simulink model "gate_V25_2016a"  (R2016a)
settings: Solver=FixedStepAuto  StartTime=0.0  StopTime=100  FixedStep=0.001  RelTol=1e-3
values from neighbouring files (symbols this model uses):
  CLOSE_CHAR = CHAR_STAR    (= 42)    [GateParameter.m]
  CLOSE_SIDE_VALUE = 2.95*oneSec    (= 2950)    [GateParameter.m]
  CLOSED = 12    [GateParameter.m]
  CLOSING = 13    [GateParameter.m]
  NO_PASS_ASSIG = 6    [GateParameter.m]
  OPEN = 14    [GateParameter.m]
  OPEN_CHAR = CHAR_HASH    (= 35)    [GateParameter.m]
  OPEN_SIDE_VALUE = 3*oneSec    (= 3000)    [GateParameter.m]
  OPEN_TIMEOUT = 60*oneSec    (= 60000)    [GateParameter.m]
  OPENING = 11    [GateParameter.m]
  OPENING_ACTIVE = 1    [GateParameter.m]
  PASS_ASSIGNED = 7    [GateParameter.m]
  PASS_INCOMPLETE = 8    [GateParameter.m]
  PASS_TIMEOUT = 10*oneSec    (= 10000)    [GateParameter.m]
  PASSWORD_VERIFIED = 5    [GateParameter.m]
  TIMEOUT = 9    [GateParameter.m]
  WRONG_PASSWORD = 2    [GateParameter.m]
undefined symbols (not defined in the file or in its folder): sigbuilder_block
libraries: simulink x9, arduinolib x4
(part 1 of 3)
settings Model: ExtModeTrigDuration=2  Creator=omaro  LastModifiedBy=oelkawok
settings OptimizationCC: DefaultParameterBehavior=Inlined  InlineInvariantSignals=on  StateBitsets=on  DataBitsets=on  LifeSpan=1  MaxStackSize=64
settings DebuggingCC: UniqueDataStoreMsg=error  StrictBusMsg=ErrorOnBusTreatedAsVector
settings HardwareCC: ProdBitPerInt=16  ProdBitPerPointer=16  ProdLargestAtomicFloat=None  ProdWordSize=8  ProdHWDeviceType=Atmel->AVR
settings SFSimCC: SimCustomHeaderCode=|
  | //#include "C:\Users\omaro\Desktop\Gate_Model\Arduino\Arduino.h"
  | //#include "Keypad\Keypad.h"
settings RTWCC: SystemTargetFile=ert.tlc  HardwareBoard=Arduino Nano 3.0  TLCOptions=-aInlineSetEventsForThisBaseRateFcn=TLC_FALSE -aSuppressMultiTaskScheduler=TLC_FALSE -aRateBasedStepFcn=1  TemplateMakefile=ert_default_tmf  GenerateReport=on  RTWUseSimCustomCode=on  Toolchain=Arduino AVR v1.6.1  BuildConfiguration=Faster Runs  LaunchReport=on
settings RTWCC: CustomHeaderCode=|
  | //#include "C:\Users\omaro\Desktop\Gate_Model\Arduino\Arduino.h"
  | //#include "Keypad\Keypad.h"
settings CodeAppCC: ForceParamTrailComments=on  OperatorAnnotations=on  MATLABSourceComments=on
settings ERTTargetCC: ERTCustomFileBanners=off  SupportContinuousTime=on  SupportNonInlinedSFcns=on  SupportVariableSizeSignals=on  ModelStepFunctionPrototypeControlCompliant=off  RootIOFormat=Structure reference

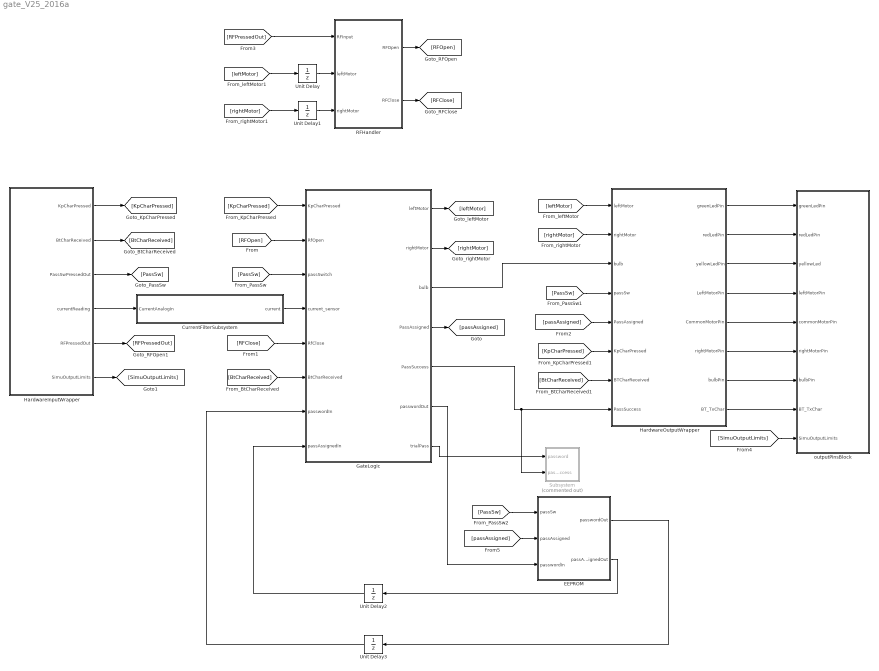
== system gate_V25_2016a ==
  CurrentFilterSubsystem : Subsystem
  EEPROM : Subsystem
  GateLogic : Subsystem  Variant=on  VariantControl=Variant1  OverrideUsingVariant=Variant2
  HardwareInputWrapper : Subsystem  Variant=on  VariantControl=Variant1  OverrideUsingVariant=Variant
  HardwareOutputWrapper : Subsystem  Variant=on  VariantControl=Variant1  OverrideUsingVariant=Variant2
  RFHandler : Subsystem
  Subsystem : Subsystem  Commented=on
  Unit Delay{,1..3} (4 alike) : UnitDelay  SampleTime=-1
  outputPinsBlock : Subsystem  Variant=on  VariantControl=Variant1  OverrideUsingVariant=Variant1
  wires:
  RFHandler/1(RFOpen) -> [RFOpen]
  RFHandler/2(RFClose) -> [RFClose]
  [RFPressedOut] -> RFHandler/1(RFInput)
  HardwareInputWrapper/5(RFPressedOut) -> [RFPressedOut]
  HardwareInputWrapper/3(PassSwPressedOut) -> [PassSw]
  [leftMotor] -> Unit Delay/1
  Unit Delay/1 -> RFHandler/2(leftMotor)
  [rightMotor] -> Unit Delay1/1
  Unit Delay1/1 -> RFHandler/3(rightMotor)
  HardwareInputWrapper/2(BtCharReceived) -> [BtCharReceived]
  HardwareInputWrapper/6(SimuOutputLimits) -> [SimuOutputLimits]
  [SimuOutputLimits] -> outputPinsBlock/9(SimuOutputLimits)
  HardwareInputWrapper/1(KpCharPressed) -> [KpCharPressed]
  [RFOpen] -> GateLogic/2(RfOpen)
  [PassSw] -> GateLogic/3(passSwitch)
  HardwareInputWrapper/4(currentReading) -> CurrentFilterSubsystem/1(CurrentAnalogIn)
  [RFClose] -> GateLogic/5(RfClose)
  [BtCharReceived] -> GateLogic/6(BtCharReceived)
  GateLogic/1(leftMotor) -> [leftMotor]
  GateLogic/2(rightMotor) -> [rightMotor]
  [KpCharPressed] -> GateLogic/1(KpCharPressed)
  [leftMotor] -> HardwareOutputWrapper/1("leftMotor ")
  [rightMotor] -> HardwareOutputWrapper/2("rightMotor ")
  GateLogic/3(bulb) -> HardwareOutputWrapper/3("bulb ")
  [PassSw] -> HardwareOutputWrapper/4("passSw ")
  [KpCharPressed] -> HardwareOutputWrapper/6("KpCharPressed ")
  [BtCharReceived] -> HardwareOutputWrapper/7("BTCharReceived ")
  HardwareOutputWrapper/1(" greenLedPin") -> outputPinsBlock/1(greenLedPin)
  HardwareOutputWrapper/2(" redLedPin") -> outputPinsBlock/2(redLedPin)
  HardwareOutputWrapper/3(" yellowLedPin") -> outputPinsBlock/3(yellowLed)
  HardwareOutputWrapper/4(" LeftMotorPin") -> outputPinsBlock/4(leftMotorPin)
  HardwareOutputWrapper/5(" CommonMotorPin") -> outputPinsBlock/5(commonMotorPin)
  HardwareOutputWrapper/6(" rightMotorPin") -> outputPinsBlock/6(rightMotorPin)
  HardwareOutputWrapper/7(" bulbPin") -> outputPinsBlock/7(bulbPin)
  HardwareOutputWrapper/8(" BT_TxChar") -> outputPinsBlock/8(BT_TxChar)
  GateLogic/4(PassAssigned) -> [passAssigned]
  [passAssigned] -> HardwareOutputWrapper/5("PassAssigned ")
  [passAssigned] -> EEPROM/2(passAssigned)
  [PassSw] -> EEPROM/1(passSw)
  GateLogic/6(passwordOut) -> EEPROM/3(passwordIn)
  EEPROM/1(passwordOut) -> Unit Delay3/1
  EEPROM/2(passAssignedOut) -> Unit Delay2/1
  Unit Delay2/1 -> GateLogic/8(passAssignedIn)
  Unit Delay3/1 -> GateLogic/7(passwordIn)
  GateLogic/5(PassSuccess) -> Subsystem/2(passSuccess), HardwareOutputWrapper/8("PassSuccess ")
  GateLogic/7(trialPass) -> Subsystem/1(password)
  CurrentFilterSubsystem/1(current) -> GateLogic/4(current_sensor)

== system gate_V25_2016a/CurrentFilterSubsystem ==
  CurrentAnalogIn : Inport
  10msSmapler : Stateflow chart  TreatAsAtomicUnit=on
      settings: PermitHierarchicalResolution=ParametersOnly
  Subsystem : Subsystem
  current : Outport
  wires:
  CurrentAnalogIn/1 -> Subsystem/1(CurrentAnalogIn)
  Subsystem/1(current) -> current/1
  10msSmapler/1(triggerOn()) -> Subsystem/Trigger

== system gate_V25_2016a/EEPROM ==
  passSw : Inport
  passAssigned : Inport  Port=2
  passwordIn : Inport  Port=3
  EEPROM_Control : Stateflow chart  TreatAsAtomicUnit=on
      settings: PermitHierarchicalResolution=ParametersOnly
  EEPROM_UPDATE : Subsystem  TreatAsAtomicUnit=on
  Subsystem2 : Subsystem  Commented=on
  Unit Delay : UnitDelay  SampleTime=-1
  Unit Delay1 : UnitDelay  SampleTime=-1
  passwordOut : Outport
  passAssignedOut : Outport  Port=2
  wires:
  passSw/1 -> EEPROM_Control/1(passSw)
  Unit Delay/1 -> EEPROM_Control/3(readComplete)
  Unit Delay1/1 -> EEPROM_Control/4(writeComplete)
  EEPROM_Control/1(clearReq) -> EEPROM_UPDATE/1(clearReq)
  EEPROM_Control/2(readReq) -> EEPROM_UPDATE/2(readReq)
  EEPROM_Control/3(writeReq) -> EEPROM_UPDATE/3(writeReq)
  passwordIn/1 -> EEPROM_UPDATE/4(passwordIn)
  [passAssigned] -> EEPROM_Control/2(passAssigned)
  [passAssigned] -> EEPROM_UPDATE/5(passAssignedIn)
  passAssigned/1 -> [passAssigned]
  EEPROM_UPDATE/1(readComplete) -> [readComplete]
  [readComplete] -> Unit Delay/1
  [writeComplete] -> Unit Delay1/1
  EEPROM_UPDATE/2(writeComplete) -> [writeComplete]
  EEPROM_UPDATE/4(passwordOut) -> passwordOut/1
  EEPROM_UPDATE/5(passAssignedOut) -> passAssignedOut/1

== system gate_V25_2016a/GateLogic ==
  KpCharPressed : Inport
  RfOpen : Inport  Port=2
  passSwitch : Inport  Port=3
  current_sensor : Inport  Port=4
  RfClose : Inport  Port=5
  BtCharReceived : Inport  Port=6
  passwordIn : Inport  Port=7
  passAssignedIn : Inport  Port=8
  A_Variant_BT_KP_RF : Subsystem  VariantControl=Variant
  B_Variant_KP_RF : Subsystem  VariantControl=Variant2
  C_Variant_RF : Subsystem  VariantControl=Variant3
  leftMotor : Outport
  rightMotor : Outport  Port=2
  bulb : Outport  Port=3
  PassAssigned : Outport  Port=4
  PassSuccess : Outport  Port=5
  passwordOut : Outport  Port=6
  trialPass : Outport  Port=7

== system gate_V25_2016a/HardwareInputWrapper ==
  HIL : Subsystem  VariantControl=Variant2
  MIL : Subsystem  VariantControl=Variant
  KpCharPressed : Outport
  BtCharReceived : Outport  Port=2
  PassSwPressedOut : Outport  Port=3
  currentReading : Outport  Port=4
  RFPressedOut : Outport  Port=5
  SimuOutputLimits : Outport  Port=6

== system gate_V25_2016a/HardwareOutputWrapper ==
  "leftMotor " : Inport
  "rightMotor " : Inport  Port=2
  "bulb " : Inport  Port=3
  "passSw " : Inport  Port=4
  "PassAssigned " : Inport  Port=5
  "KpCharPressed " : Inport  Port=6
  "BTCharReceived " : Inport  Port=7
  "PassSuccess " : Inport  Port=8
  A_HardwareOutputWrapper_BT_KP_RF : Subsystem  VariantControl=Variant1
  B_HardwareOutputWrapper_KP_RF : Subsystem  VariantControl=Variant2
  C_HardwareOutputWrapper_RF : Subsystem  VariantControl=Variant3
  " greenLedPin" : Outport
  " redLedPin" : Outport  Port=2
  " yellowLedPin" : Outport  Port=3
  " LeftMotorPin" : Outport  Port=4
  " CommonMotorPin" : Outport  Port=5
  " rightMotorPin" : Outport  Port=6
  " bulbPin" : Outport  Port=7
  " BT_TxChar" : Outport  Port=8

== system gate_V25_2016a/RFHandler ==
  RFInput : Inport
  leftMotor : Inport  Port=2
  rightMotor : Inport  Port=3
  CLOSED : Constant  Value=CLOSED  SampleTime=-1
  CLOSING : Constant  Value=CLOSING  SampleTime=-1
  OPEN : Constant  Value=OPEN  SampleTime=-1
  OPENING : Constant  Value=OPENING  SampleTime=-1
  RFHandlerL : Stateflow chart  TreatAsAtomicUnit=on
      settings: PermitHierarchicalResolution=ParametersOnly
  Scope : Scope
  RFOpen : Outport
  RFClose : Outport  Port=2
  wires:
  RFInput/1 -> RFHandlerL/1(btn)
  RFHandlerL/1(RFClose) -> RFClose/1
  RFHandlerL/2(RFOpen) -> Scope/1, RFOpen/1
  OPEN/1 -> RFHandlerL/6(OPEN)
  CLOSING/1 -> RFHandlerL/5(CLOSING)
  CLOSED/1 -> RFHandlerL/4(CLOSED)
  OPENING/1 -> RFHandlerL/7(OPENING)
  leftMotor/1 -> RFHandlerL/2(leftMotor)
  rightMotor/1 -> RFHandlerL/3(rightMotor)

== system gate_V25_2016a/Subsystem ==
  password : Inport
  passSuccess : Inport  Port=2
  S-Function Builder1 : S-Function  Commented=on  InitFcn=try, set_param(gcb,'FunctionName','printingBlock'), end  FunctionName=printingBlock  SFunctionModules=printingBlock_wrapper  SFunctionDeploymentMode=off  EnableBusSupport=off  mask(S-Function Builder){}
      mask help: Simulink:masks:SFunctionBuilder_MD
      mask init:
      | val = [[.9  0.75 0.75 1 1 .9 .9 1]',[1 1 0.75 0.75 .9 .9 1 .9]'];try , sys = get_param(gcb,'SfunBuilderFcnName');if isempty(sys), sys = get_param(gcb,'FunctionName'); end,catch, sys = get_param(gcb,'FunctionName'); end
      settings: CopyFcn=set_param(gcbh,'LinkStatus','none')  PreSaveFcn=try, set_param(gcb,'FunctionName','printingBlock'), end  OpenFcn=sfunctionwizard(gcbh)
      mask Display: plot(val(:,1),val(:,2)),disp(sys), port_label('input',1,'input'), port_label('input',2,'oldInput')
  S-Function Builder2 : S-Function  InitFcn=try, set_param(gcb,'FunctionName','printingPassBlock'), end  FunctionName=printingPassBlock  SFunctionModules=printingPassBlock_wrapper  SFunctionDeploymentMode=off  EnableBusSupport=off  mask(S-Function Builder){}
      mask help: Simulink:masks:SFunctionBuilder_MD
      mask init: same as gate_V25_2016a/Subsystem/S-Function Builder1
      settings: CopyFcn=set_param(gcbh,'LinkStatus','none')  PreSaveFcn=try, set_param(gcb,'FunctionName','printingPassBlock'), end  OpenFcn=sfunctionwizard(gcbh)
      mask Display: plot(val(:,1),val(:,2)),disp(sys), port_label('input',1,'password'), port_label('input',2,'passSuccess')
  wires:
  password/1 -> S-Function Builder2/1
  passSuccess/1 -> S-Function Builder2/2

== system gate_V25_2016a/outputPinsBlock ==
  greenLedPin : Inport
  redLedPin : Inport  Port=2
  yellowLed : Inport  Port=3
  leftMotorPin : Inport  Port=4
  commonMotorPin : Inport  Port=5
  rightMotorPin : Inport  Port=6
  bulbPin : Inport  Port=7
  BT_TxChar : Inport  Port=8
  SimuOutputLimits : Inport  Port=9
  HIL : Subsystem  VariantControl=Variant
  MIL : Subsystem  Variant=on  VariantControl=Variant1  OverrideUsingVariant=Variant1

== system gate_V25_2016a/CurrentFilterSubsystem/Subsystem ==
  CurrentAnalogIn : Inport
  Trigger : TriggerPort  TriggerType=function-call  VariantControl=Variant  PortDimensions=1
  Scope : Scope
  SquareWaveDetector : Stateflow chart  TreatAsAtomicUnit=on
      settings: PermitHierarchicalResolution=ParametersOnly
  Unit Delay : UnitDelay  SampleTime=-1
  current : Outport
  wires:
  Unit Delay/1 -> SquareWaveDetector/2(CurrentAnalogInOld)
  CurrentAnalogIn/1 -> Unit Delay/1, SquareWaveDetector/1(CurrentAnalogIn)
  SquareWaveDetector/1(currentValue) -> current/1, Scope/1

== system gate_V25_2016a/EEPROM/EEPROM_UPDATE ==
  clearReq : Inport
  readReq : Inport  Port=2
  writeReq : Inport  Port=3
  passwordIn : Inport  Port=4
  passAssignedIn : Inport  Port=5
  S-Function Builder : S-Function  InitFcn=try, set_param(gcb,'FunctionName','myEEPROM_Handler'), end  FunctionName=myEEPROM_Handler  SFunctionModules=myEEPROM_Handler_wrapper  SFunctionDeploymentMode=off  EnableBusSupport=off  mask(S-Function Builder){}
      mask help: Simulink:masks:SFunctionBuilder_MD
      mask init: same as gate_V25_2016a/Subsystem/S-Function Builder1
      settings: CopyFcn=set_param(gcbh,'LinkStatus','none')  PreSaveFcn=try, set_param(gcb,'FunctionName','myEEPROM_Handler'), end  OpenFcn=sfunctionwizard(gcbh)
      mask Display: plot(val(:,1),val(:,2)),disp(sys), port_label('input',1,'passwordIn'), port_label('input',2,'readReq'), port_label('input',3,'oldReadReq'), port_label('input',4,'clearReq'), port_label('input',5,'oldClearReq'), port_label('input',6,'writeReq'), port_label('input',7,'oldWriteReq'), port_label('input',8,'passAssignedIn'), port_label('output',1,'passwordOut'), port_label('output',2,'readComplete'), port_label('output',3,'writeComplete'), port_label('output',4,'clearComplete'), port_label('output',5,'passAssignedOut')
  Unit Delay : UnitDelay  SampleTime=-1
  Unit Delay1 : UnitDelay  SampleTime=-1
  Unit Delay2 : UnitDelay  SampleTime=-1
  readComplete : Outport
  writeComplete : Outport  Port=2
  clearComplete : Outport  Port=3
  passwordOut : Outport  Port=4
  passAssignedOut : Outport  Port=5
  wires:
  S-Function Builder/3 -> writeComplete/1
  S-Function Builder/2 -> readComplete/1
  S-Function Builder/4 -> clearComplete/1
  passwordIn/1 -> S-Function Builder/1
  readReq/1 -> Unit Delay/1, S-Function Builder/2
  Unit Delay/1 -> S-Function Builder/3
  clearReq/1 -> Unit Delay1/1, S-Function Builder/4
  passAssignedIn/1 -> S-Function Builder/8
  writeReq/1 -> Unit Delay2/1, S-Function Builder/6
  Unit Delay2/1 -> S-Function Builder/7
  Unit Delay1/1 -> S-Function Builder/5
  S-Function Builder/1 -> passwordOut/1
  S-Function Builder/5 -> passAssignedOut/1

== system gate_V25_2016a/EEPROM/Subsystem2 ==
  clearReq : Inport
  readReq : Inport  Port=2
  writeReq : Inport  Port=3
  passwordIn : Inport  Port=4
  passAssignedIn : Inport  Port=5
  S-Function Builder : S-Function  InitFcn=try, set_param(gcb,'FunctionName','EEPROM_Handler'), end  FunctionName=EEPROM_Handler  SFunctionModules=EEPROM_Handler_wrapper  SFunctionDeploymentMode=off  EnableBusSupport=off  mask(S-Function Builder){}
      mask help: Simulink:masks:SFunctionBuilder_MD
      mask init: same as gate_V25_2016a/Subsystem/S-Function Builder1
      settings: CopyFcn=set_param(gcbh,'LinkStatus','none')  PreSaveFcn=try, set_param(gcb,'FunctionName','EEPROM_Handler'), end  OpenFcn=sfunctionwizard(gcbh)
      mask Display:
      | plot(val(:,1),val(:,2))
      | disp(sys)
      | port_label('input',1,'passwordIn')
      | port_label('input',2,'readReq')
      | port_label('input',3,'clearReq')
      | port_label('input',4,'writeReq')
      | port_label('input',5,'passAssignedIn')
      | port_label('output',1,'passwordOut')
      | port_label('output',2,'readComplete')
      | port_label('output',3,'writeComplete')
      | port_label('output',4,'clearComplete')
      | port_label('output',5,'passAssignedOut')
  Scope3 : Scope  NumInputPorts=5
  readComplete : Outport
  writeComplete : Outport  Port=2
  clearComplete : Outport  Port=3
  passwordOut : Outport  Port=4
  passAssignedOut : Outport  Port=5
  wires:
  S-Function Builder/5 -> passAssignedOut/1, Scope3/5
  S-Function Builder/3 -> writeComplete/1, Scope3/3
  S-Function Builder/2 -> readComplete/1, Scope3/2
  S-Function Builder/1 -> passwordOut/1, Scope3/1
  S-Function Builder/4 -> clearComplete/1, Scope3/4
  passAssignedIn/1 -> S-Function Builder/5
  clearReq/1 -> S-Function Builder/3
  passwordIn/1 -> S-Function Builder/1
  readReq/1 -> S-Function Builder/2
  writeReq/1 -> S-Function Builder/4

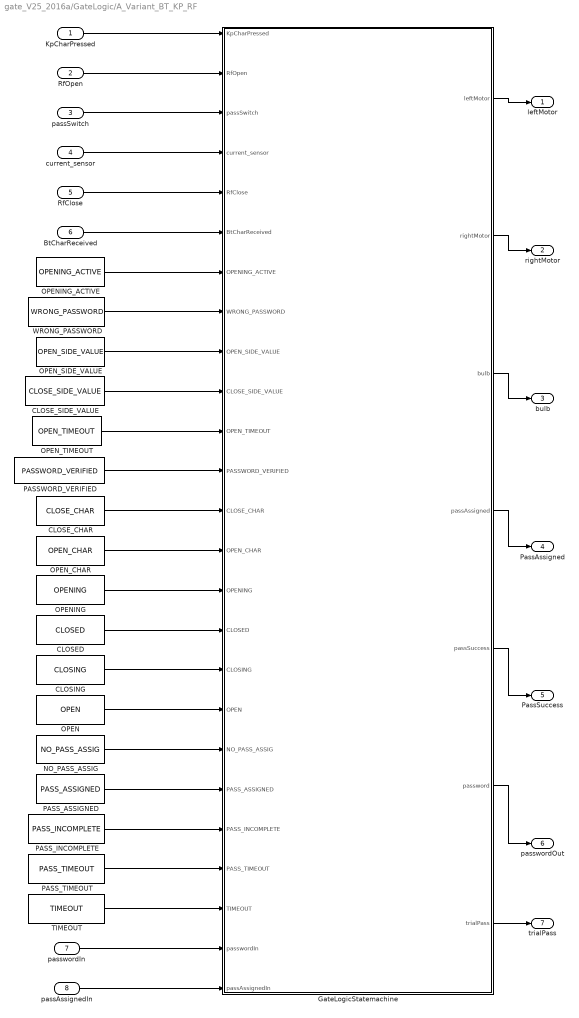
== system gate_V25_2016a/GateLogic/A_Variant_BT_KP_RF ==
  KpCharPressed : Inport
  RfOpen : Inport  Port=2
  passSwitch : Inport  Port=3
  current_sensor : Inport  Port=4
  RfClose : Inport  Port=5
  BtCharReceived : Inport  Port=6
  passwordIn : Inport  Port=7
  passAssignedIn : Inport  Port=8
  CLOSED : Constant  Value=CLOSED  SampleTime=-1
  CLOSE_CHAR : Constant  Value=CLOSE_CHAR  SampleTime=-1
  CLOSE_SIDE_VALUE : Constant  Value=CLOSE_SIDE_VALUE  SampleTime=-1
  CLOSING : Constant  Value=CLOSING  SampleTime=-1
  GateLogicStatemachine : Stateflow chart  TreatAsAtomicUnit=on
      settings: PermitHierarchicalResolution=ParametersOnly
  NO_PASS_ASSIG : Constant  Value=NO_PASS_ASSIG  SampleTime=-1
  OPEN : Constant  Value=OPEN  SampleTime=-1
  OPENING : Constant  Value=OPENING  SampleTime=-1
  OPENING_ACTIVE : Constant  Value=OPENING_ACTIVE  SampleTime=-1
  OPEN_CHAR : Constant  Value=OPEN_CHAR  SampleTime=-1
  OPEN_SIDE_VALUE : Constant  Value=OPEN_SIDE_VALUE  SampleTime=-1
  OPEN_TIMEOUT : Constant  Value=OPEN_TIMEOUT  SampleTime=-1
  PASSWORD_VERIFIED : Constant  Value=PASSWORD_VERIFIED  SampleTime=-1
  PASS_ASSIGNED : Constant  Value=PASS_ASSIGNED  SampleTime=-1
  PASS_INCOMPLETE : Constant  Value=PASS_INCOMPLETE  SampleTime=-1
  PASS_TIMEOUT : Constant  Value=PASS_TIMEOUT  SampleTime=-1
  TIMEOUT : Constant  Value=TIMEOUT  SampleTime=-1
  WRONG_PASSWORD : Constant  Value=WRONG_PASSWORD  SampleTime=-1
  leftMotor : Outport
  rightMotor : Outport  Port=2
  bulb : Outport  Port=3
  PassAssigned : Outport  Port=4
  PassSuccess : Outport  Port=5
  passwordOut : Outport  Port=6
  trialPass : Outport  Port=7
  wires:
  RfClose/1 -> GateLogicStatemachine/5(RfClose)
  TIMEOUT/1 -> GateLogicStatemachine/23(TIMEOUT)
  PASS_INCOMPLETE/1 -> GateLogicStatemachine/21(PASS_INCOMPLETE)
  PASS_ASSIGNED/1 -> GateLogicStatemachine/20(PASS_ASSIGNED)
  GateLogicStatemachine/4(passAssigned) -> PassAssigned/1
  passSwitch/1 -> GateLogicStatemachine/3(passSwitch)
  GateLogicStatemachine/5(passSuccess) -> PassSuccess/1
  PASS_TIMEOUT/1 -> GateLogicStatemachine/22(PASS_TIMEOUT)
  KpCharPressed/1 -> GateLogicStatemachine/1(KpCharPressed)
  BtCharReceived/1 -> GateLogicStatemachine/6(BtCharReceived)
  NO_PASS_ASSIG/1 -> GateLogicStatemachine/19(NO_PASS_ASSIG)
  CLOSE_SIDE_VALUE/1 -> GateLogicStatemachine/10(CLOSE_SIDE_VALUE)
  OPEN_TIMEOUT/1 -> GateLogicStatemachine/11(OPEN_TIMEOUT)
  OPEN_SIDE_VALUE/1 -> GateLogicStatemachine/9(OPEN_SIDE_VALUE)
  OPENING_ACTIVE/1 -> GateLogicStatemachine/7(OPENING_ACTIVE)
  GateLogicStatemachine/2(rightMotor) -> rightMotor/1
  GateLogicStatemachine/1(leftMotor) -> leftMotor/1
  WRONG_PASSWORD/1 -> GateLogicStatemachine/8(WRONG_PASSWORD)
  current_sensor/1 -> GateLogicStatemachine/4(current_sensor)
  GateLogicStatemachine/3(bulb) -> bulb/1
  RfOpen/1 -> GateLogicStatemachine/2(RfOpen)
  PASSWORD_VERIFIED/1 -> GateLogicStatemachine/12(PASSWORD_VERIFIED)
  OPEN/1 -> GateLogicStatemachine/18(OPEN)
  CLOSE_CHAR/1 -> GateLogicStatemachine/13(CLOSE_CHAR)
  OPEN_CHAR/1 -> GateLogicStatemachine/14(OPEN_CHAR)
  CLOSED/1 -> GateLogicStatemachine/16(CLOSED)
  OPENING/1 -> GateLogicStatemachine/15(OPENING)
  CLOSING/1 -> GateLogicStatemachine/17(CLOSING)
  GateLogicStatemachine/6(password) -> passwordOut/1
  passwordIn/1 -> GateLogicStatemachine/24(passwordIn)
  passAssignedIn/1 -> GateLogicStatemachine/25(passAssignedIn)
  GateLogicStatemachine/7(trialPass) -> trialPass/1

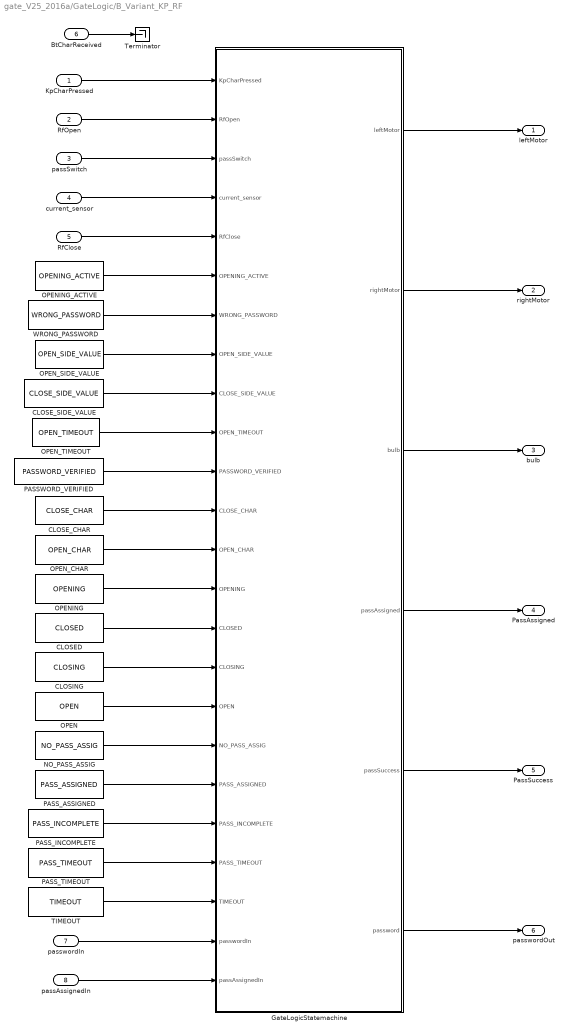
== system gate_V25_2016a/GateLogic/B_Variant_KP_RF ==
  KpCharPressed : Inport
  RfOpen : Inport  Port=2
  passSwitch : Inport  Port=3
  current_sensor : Inport  Port=4
  RfClose : Inport  Port=5
  BtCharReceived : Inport  Port=6
  passwordIn : Inport  Port=7
  passAssignedIn : Inport  Port=8
  CLOSED : Constant  Value=CLOSED  SampleTime=-1
  CLOSE_CHAR : Constant  Value=CLOSE_CHAR  SampleTime=-1
  CLOSE_SIDE_VALUE : Constant  Value=CLOSE_SIDE_VALUE  SampleTime=-1
  CLOSING : Constant  Value=CLOSING  SampleTime=-1
  GateLogicStatemachine : Stateflow chart  TreatAsAtomicUnit=on
      settings: PermitHierarchicalResolution=ParametersOnly
  NO_PASS_ASSIG : Constant  Value=NO_PASS_ASSIG  SampleTime=-1
  OPEN : Constant  Value=OPEN  SampleTime=-1
  OPENING : Constant  Value=OPENING  SampleTime=-1
  OPENING_ACTIVE : Constant  Value=OPENING_ACTIVE  SampleTime=-1
  OPEN_CHAR : Constant  Value=OPEN_CHAR  SampleTime=-1
  OPEN_SIDE_VALUE : Constant  Value=OPEN_SIDE_VALUE  SampleTime=-1
  OPEN_TIMEOUT : Constant  Value=OPEN_TIMEOUT  SampleTime=-1
  PASSWORD_VERIFIED : Constant  Value=PASSWORD_VERIFIED  SampleTime=-1
  PASS_ASSIGNED : Constant  Value=PASS_ASSIGNED  SampleTime=-1
  PASS_INCOMPLETE : Constant  Value=PASS_INCOMPLETE  SampleTime=-1
  PASS_TIMEOUT : Constant  Value=PASS_TIMEOUT  SampleTime=-1
  TIMEOUT : Constant  Value=TIMEOUT  SampleTime=-1
  Terminator : Terminator
  WRONG_PASSWORD : Constant  Value=WRONG_PASSWORD  SampleTime=-1
  leftMotor : Outport
  rightMotor : Outport  Port=2
  bulb : Outport  Port=3
  PassAssigned : Outport  Port=4
  PassSuccess : Outport  Port=5
  passwordOut : Outport  Port=6
  wires:
  CLOSING/1 -> GateLogicStatemachine/16(CLOSING)
  OPENING/1 -> GateLogicStatemachine/14(OPENING)
  CLOSED/1 -> GateLogicStatemachine/15(CLOSED)
  OPEN_CHAR/1 -> GateLogicStatemachine/13(OPEN_CHAR)
  CLOSE_CHAR/1 -> GateLogicStatemachine/12(CLOSE_CHAR)
  OPEN/1 -> GateLogicStatemachine/17(OPEN)
  PASSWORD_VERIFIED/1 -> GateLogicStatemachine/11(PASSWORD_VERIFIED)
  RfOpen/1 -> GateLogicStatemachine/2(RfOpen)
  GateLogicStatemachine/3(bulb) -> bulb/1
  current_sensor/1 -> GateLogicStatemachine/4(current_sensor)
  WRONG_PASSWORD/1 -> GateLogicStatemachine/7(WRONG_PASSWORD)
  GateLogicStatemachine/1(leftMotor) -> leftMotor/1
  GateLogicStatemachine/2(rightMotor) -> rightMotor/1
  OPENING_ACTIVE/1 -> GateLogicStatemachine/6(OPENING_ACTIVE)
  OPEN_SIDE_VALUE/1 -> GateLogicStatemachine/8(OPEN_SIDE_VALUE)
  OPEN_TIMEOUT/1 -> GateLogicStatemachine/10(OPEN_TIMEOUT)
  CLOSE_SIDE_VALUE/1 -> GateLogicStatemachine/9(CLOSE_SIDE_VALUE)
  NO_PASS_ASSIG/1 -> GateLogicStatemachine/18(NO_PASS_ASSIG)
  KpCharPressed/1 -> GateLogicStatemachine/1(KpCharPressed)
  PASS_TIMEOUT/1 -> GateLogicStatemachine/21(PASS_TIMEOUT)
  GateLogicStatemachine/5(passSuccess) -> PassSuccess/1
  passSwitch/1 -> GateLogicStatemachine/3(passSwitch)
  GateLogicStatemachine/4(passAssigned) -> PassAssigned/1
  PASS_ASSIGNED/1 -> GateLogicStatemachine/19(PASS_ASSIGNED)
  PASS_INCOMPLETE/1 -> GateLogicStatemachine/20(PASS_INCOMPLETE)
  TIMEOUT/1 -> GateLogicStatemachine/22(TIMEOUT)
  RfClose/1 -> GateLogicStatemachine/5(RfClose)
  BtCharReceived/1 -> Terminator/1
  passwordIn/1 -> GateLogicStatemachine/23(passwordIn)
  passAssignedIn/1 -> GateLogicStatemachine/24(passAssignedIn)
  GateLogicStatemachine/6(password) -> passwordOut/1

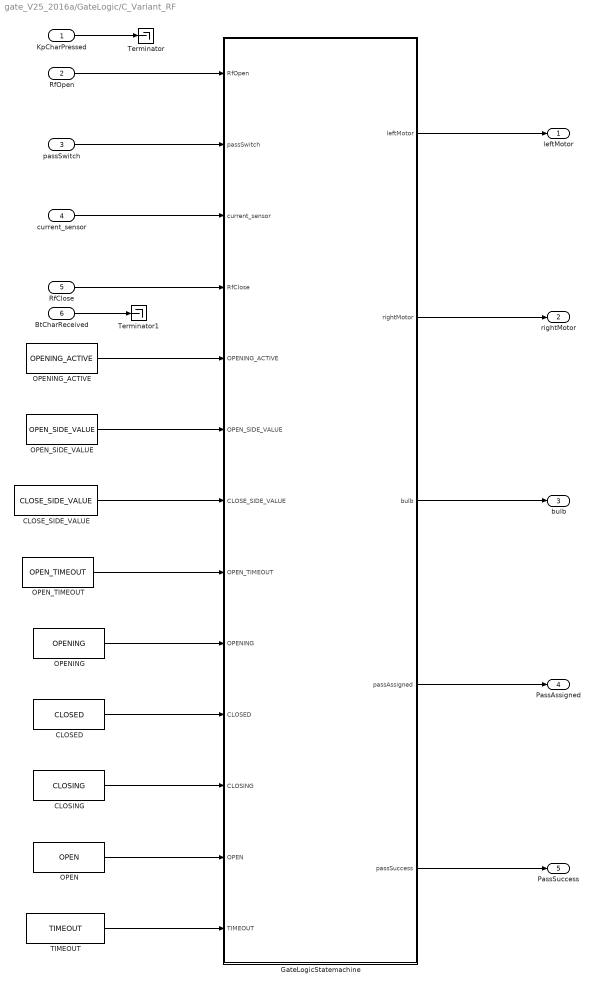
== system gate_V25_2016a/GateLogic/C_Variant_RF ==
  KpCharPressed : Inport
  RfOpen : Inport  Port=2
  passSwitch : Inport  Port=3
  current_sensor : Inport  Port=4
  RfClose : Inport  Port=5
  BtCharReceived : Inport  Port=6
  CLOSED : Constant  Value=CLOSED  SampleTime=-1
  CLOSE_SIDE_VALUE : Constant  Value=CLOSE_SIDE_VALUE  SampleTime=-1
  CLOSING : Constant  Value=CLOSING  SampleTime=-1
  GateLogicStatemachine : Stateflow chart  TreatAsAtomicUnit=on
      settings: PermitHierarchicalResolution=ParametersOnly
  OPEN : Constant  Value=OPEN  SampleTime=-1
  OPENING : Constant  Value=OPENING  SampleTime=-1
  OPENING_ACTIVE : Constant  Value=OPENING_ACTIVE  SampleTime=-1
  OPEN_SIDE_VALUE : Constant  Value=OPEN_SIDE_VALUE  SampleTime=-1
  OPEN_TIMEOUT : Constant  Value=OPEN_TIMEOUT  SampleTime=-1
  TIMEOUT : Constant  Value=TIMEOUT  SampleTime=-1
  Terminator : Terminator
  Terminator1 : Terminator
  leftMotor : Outport
  rightMotor : Outport  Port=2
  bulb : Outport  Port=3
  PassAssigned : Outport  Port=4
  PassSuccess : Outport  Port=5
  wires:
  RfClose/1 -> GateLogicStatemachine/4(RfClose)
  TIMEOUT/1 -> GateLogicStatemachine/13(TIMEOUT)
  GateLogicStatemachine/4(passAssigned) -> PassAssigned/1
  passSwitch/1 -> GateLogicStatemachine/2(passSwitch)
  GateLogicStatemachine/5(passSuccess) -> PassSuccess/1
  CLOSE_SIDE_VALUE/1 -> GateLogicStatemachine/7(CLOSE_SIDE_VALUE)
  OPEN_TIMEOUT/1 -> GateLogicStatemachine/8(OPEN_TIMEOUT)
  OPEN_SIDE_VALUE/1 -> GateLogicStatemachine/6(OPEN_SIDE_VALUE)
  OPENING_ACTIVE/1 -> GateLogicStatemachine/5(OPENING_ACTIVE)
  GateLogicStatemachine/2(rightMotor) -> rightMotor/1
  GateLogicStatemachine/1(leftMotor) -> leftMotor/1
  current_sensor/1 -> GateLogicStatemachine/3(current_sensor)
  GateLogicStatemachine/3(bulb) -> bulb/1
  RfOpen/1 -> GateLogicStatemachine/1(RfOpen)
  OPEN/1 -> GateLogicStatemachine/12(OPEN)
  CLOSED/1 -> GateLogicStatemachine/10(CLOSED)
  OPENING/1 -> GateLogicStatemachine/9(OPENING)
  CLOSING/1 -> GateLogicStatemachine/11(CLOSING)
  KpCharPressed/1 -> Terminator/1
  BtCharReceived/1 -> Terminator1/1

== system gate_V25_2016a/HardwareInputWrapper/HIL ==
  Analog Input : arduinolib/Analog Input  pinNumber=6  sampleTime=-1  blockPlatform=arduino
  BluetoothWrapper : Subsystem
  ButtonsPressed : Subsystem
  KeypadWrapper : Subsystem
  S-Function Builder1 : S-Function  Commented=on  InitFcn=try, set_param(gcb,'FunctionName','CurrentA_Lib'), end  FunctionName=CurrentA_Lib  SFunctionModules=CurrentA_Lib_wrapper  SFunctionDeploymentMode=off  EnableBusSupport=off  mask(S-Function Builder){}
      mask help: Simulink:masks:SFunctionBuilder_MD
      mask init: same as gate_V25_2016a/Subsystem/S-Function Builder1
      settings: CopyFcn=set_param(gcbh,'LinkStatus','none')  PreSaveFcn=try, set_param(gcb,'FunctionName','CurrentA_Lib'), end  OpenFcn=sfunctionwizard(gcbh)
      mask Display: plot(val(:,1),val(:,2)),disp(sys), port_label('output',1,'currentValue')
  S-Function Builder2 : S-Function  Commented=on  InitFcn=try, set_param(gcb,'FunctionName','printingBlock'), end  FunctionName=printingBlock  SFunctionModules=printingBlock_wrapper  SFunctionDeploymentMode=off  EnableBusSupport=off  mask(S-Function Builder){}
      mask help: Simulink:masks:SFunctionBuilder_MD
      mask init: same as gate_V25_2016a/Subsystem/S-Function Builder1
      settings: CopyFcn=set_param(gcbh,'LinkStatus','none')  PreSaveFcn=try, set_param(gcb,'FunctionName','printingBlock'), end  OpenFcn=sfunctionwizard(gcbh)
      mask Display: plot(val(:,1),val(:,2)),disp(sys), port_label('input',1,'uint8ToPrint')
  currentSensorWrapperOld : Subsystem  Commented=on
  KpCharPressed : Outport
  BtCharReceived : Outport  Port=2
  PassSwPressedOut : Outport  Port=3
  currentReading : Outport  Port=4
  RFPressedOut : Outport  Port=5
  wires:
  BluetoothWrapper/1(bluetoothCharPressed) -> BtCharReceived/1
  Analog Input/1 -> currentReading/1  "motorCrrent"
  KeypadWrapper/1(charPressed) -> S-Function Builder2/1, KpCharPressed/1
  ButtonsPressed/2(SWPressed) -> PassSwPressedOut/1
  ButtonsPressed/1(RFPressed) -> RFPressedOut/1

== system gate_V25_2016a/HardwareInputWrapper/MIL ==
  Bus Creator : BusCreator  Inputs=16
  Quantizer{,1..3} (4 alike) : Quantizer  QuantizationInterval=-1
  Signal Builder : Subsystem  Tag=STV Subsys  LoadFcn=sigbuilder_block('load');  StartFcn=sigbuilder_block('start');  StopFcn=sigbuilder_block('stop');  ClipboardFcn=sigbuilder_block('clipboard');  mask(Sigbuilder block){}
      mask help: Simulink:masks:SigbuilderBlock_MD
      mask init:
      | if ~strcmp(get_param(bdroot(gcbh),'SimulationStatus'),'stopped') tuvar = sigbuilder_block('maskInit'); end
      settings: CopyFcn=sigbuilder_block('copy');  DeleteFcn=sigbuilder_block('delete');  ModelCloseFcn=sigbuilder_block('modelClose');  PreSaveFcn=sigbuilder_block('preSave');  PauseFcn=sigbuilder_block('pause');  ContinueFcn=sigbuilder_block('continue');  NameChangeFcn=sigbuilder_block('namechange');  OpenFcn=sigbuilder_block('open',[6 28.2 1012.8 484.8 ]);  CloseFcn=sigbuilder_block('close');
      mask Display: plot(0, 0, 100, 100,[2, 2, 32, 32, 2], [68, 8, 8, 68, 68],[32, 2], [38, 38], [32, 19, 2],[53, 60, 44], [32, 17, 17, 2],[16, 16, 31, 31]);txt = getActiveGroup(gcbh);text(2, 100, txt,'verticalAlignment', 'top');
  KpCharPressed : Outport
  BtCharReceived : Outport  Port=2
  PassSwPressedOut : Outport  Port=3
  RFPressedOut : Outport  Port=4
  currentReading : Outport  Port=5
  SimuOutputLimits : Outport  Port=6
  wires:
  Signal Builder/2(BT_input) -> Quantizer1/1
  Signal Builder/4(SW_input) -> Quantizer3/1
  Signal Builder/1(Kp_input) -> Quantizer/1
  Signal Builder/3(RF_input) -> Quantizer2/1
  Quantizer/1 -> KpCharPressed/1
  Quantizer1/1 -> BtCharReceived/1
  Quantizer2/1 -> RFPressedOut/1
  Quantizer3/1 -> PassSwPressedOut/1
  Bus Creator/1 -> SimuOutputLimits/1
  Signal Builder/16(GreenLedMax) -> Bus Creator/11  "GreenLedMax"
  Signal Builder/15(YellowLedMin) -> Bus Creator/10  "YellowLedMin"
  Signal Builder/17(GreenLedMin) -> Bus Creator/12  "GreenLedMin"
  Signal Builder/14(YellowLedMax) -> Bus Creator/9  "YellowLedMax"
  Signal Builder/18(BulbMax) -> Bus Creator/13  "BulbMax"
  Signal Builder/13(RedLedMin) -> Bus Creator/8  "RedLedMin"
  Signal Builder/19(BulbMin) -> Bus Creator/14  "BulbMin"
  Signal Builder/20(BT_outputMax) -> Bus Creator/15  "BT_outputMax"
  Signal Builder/12(RedLedMax) -> Bus Creator/7  "RedLedMax"
  Signal Builder/11(MCMin) -> Bus Creator/6  "MCMin"
  Signal Builder/10(MCMax) -> Bus Creator/5  "MCMax"
  Signal Builder/9(MRMin) -> Bus Creator/4  "MRMin"
  Signal Builder/8(MRMax) -> Bus Creator/3  "MRMax"
  Signal Builder/7(MLMin) -> Bus Creator/2  "MLMin"
  Signal Builder/6(MLMax) -> Bus Creator/1  "MLMax"
  Signal Builder/21(BT_outputMin) -> Bus Creator/16  "BT_outputMin"
  Signal Builder/5(currentReading_input) -> currentReading/1

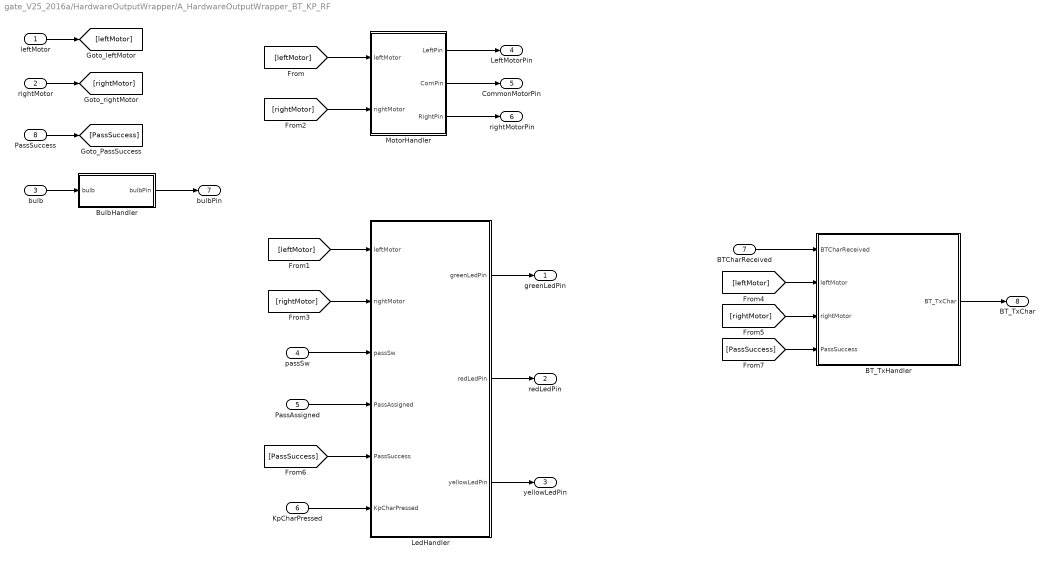
== system gate_V25_2016a/HardwareOutputWrapper/A_HardwareOutputWrapper_BT_KP_RF ==
  leftMotor : Inport
  rightMotor : Inport  Port=2
  bulb : Inport  Port=3
  passSw : Inport  Port=4
  PassAssigned : Inport  Port=5
  KpCharPressed : Inport  Port=6
  BTCharReceived : Inport  Port=7
  PassSuccess : Inport  Port=8
  BT_TxHandler : Subsystem
  BulbHandler : Subsystem
  LedHandler : Subsystem
  MotorHandler : Subsystem
  greenLedPin : Outport
  redLedPin : Outport  Port=2
  yellowLedPin : Outport  Port=3
  LeftMotorPin : Outport  Port=4
  CommonMotorPin : Outport  Port=5
  rightMotorPin : Outport  Port=6
  bulbPin : Outport  Port=7
  BT_TxChar : Outport  Port=8
  wires:
  [leftMotor] -> MotorHandler/1(leftMotor)
  [rightMotor] -> MotorHandler/2(rightMotor)
  bulb/1 -> BulbHandler/1(bulb)
  LedHandler/1(greenLedPin) -> greenLedPin/1
  LedHandler/2(redLedPin) -> redLedPin/1
  LedHandler/3(yellowLedPin) -> yellowLedPin/1
  MotorHandler/1(LeftPin) -> LeftMotorPin/1
  MotorHandler/2(ComPin) -> CommonMotorPin/1
  MotorHandler/3(RightPin) -> rightMotorPin/1
  BulbHandler/1(bulbPin) -> bulbPin/1
  leftMotor/1 -> [leftMotor]
  [leftMotor] -> LedHandler/1(leftMotor)
  rightMotor/1 -> [rightMotor]
  [rightMotor] -> LedHandler/2(rightMotor)
  passSw/1 -> LedHandler/3(passSw)
  PassAssigned/1 -> LedHandler/4(PassAssigned)
  [PassSuccess] -> LedHandler/5(PassSuccess)
  KpCharPressed/1 -> LedHandler/6(KpCharPressed)
  [leftMotor] -> BT_TxHandler/2(leftMotor)
  BTCharReceived/1 -> BT_TxHandler/1(BTCharReceived)
  [rightMotor] -> BT_TxHandler/3(rightMotor)
  PassSuccess/1 -> [PassSuccess]
  [PassSuccess] -> BT_TxHandler/4(PassSuccess)
  BT_TxHandler/1(BT_TxChar) -> BT_TxChar/1

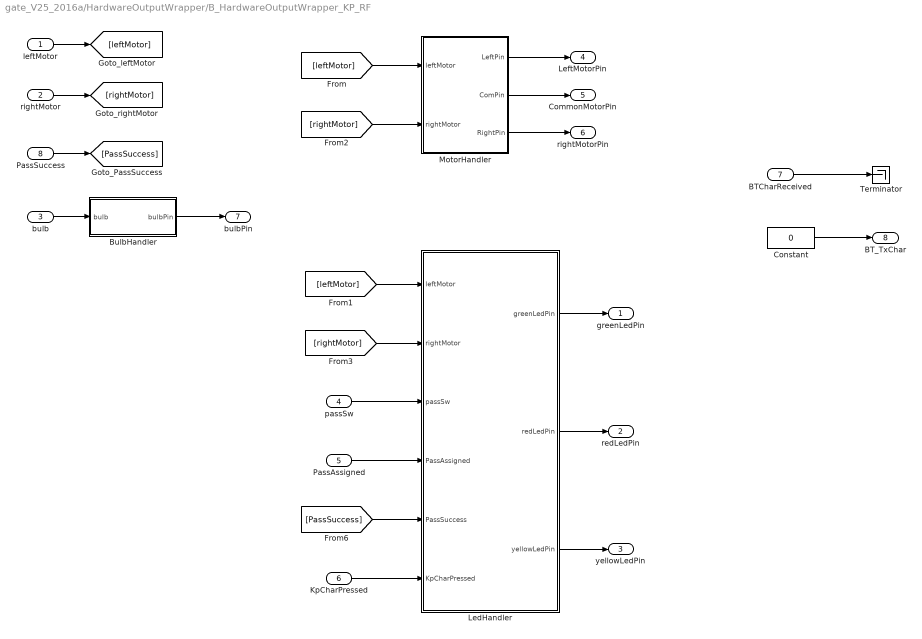
== system gate_V25_2016a/HardwareOutputWrapper/B_HardwareOutputWrapper_KP_RF ==
  leftMotor : Inport
  rightMotor : Inport  Port=2
  bulb : Inport  Port=3
  passSw : Inport  Port=4
  PassAssigned : Inport  Port=5
  KpCharPressed : Inport  Port=6
  BTCharReceived : Inport  Port=7
  PassSuccess : Inport  Port=8
  BulbHandler : Subsystem
  Constant : Constant  Value=0  SampleTime=-1
  LedHandler : Subsystem
  MotorHandler : Subsystem
  Terminator : Terminator
  greenLedPin : Outport
  redLedPin : Outport  Port=2
  yellowLedPin : Outport  Port=3
  LeftMotorPin : Outport  Port=4
  CommonMotorPin : Outport  Port=5
  rightMotorPin : Outport  Port=6
  bulbPin : Outport  Port=7
  BT_TxChar : Outport  Port=8
  wires:
  Constant/1 -> BT_TxChar/1
  PassSuccess/1 -> [PassSuccess]
  KpCharPressed/1 -> LedHandler/6(KpCharPressed)
  [PassSuccess] -> LedHandler/5(PassSuccess)
  PassAssigned/1 -> LedHandler/4(PassAssigned)
  passSw/1 -> LedHandler/3(passSw)
  [rightMotor] -> LedHandler/2(rightMotor)
  rightMotor/1 -> [rightMotor]
  [leftMotor] -> LedHandler/1(leftMotor)
  leftMotor/1 -> [leftMotor]
  BulbHandler/1(bulbPin) -> bulbPin/1
  MotorHandler/3(RightPin) -> rightMotorPin/1
  MotorHandler/2(ComPin) -> CommonMotorPin/1
  MotorHandler/1(LeftPin) -> LeftMotorPin/1
  LedHandler/3(yellowLedPin) -> yellowLedPin/1
  LedHandler/2(redLedPin) -> redLedPin/1
  LedHandler/1(greenLedPin) -> greenLedPin/1
  bulb/1 -> BulbHandler/1(bulb)
  [rightMotor] -> MotorHandler/2(rightMotor)
  [leftMotor] -> MotorHandler/1(leftMotor)
  BTCharReceived/1 -> Terminator/1

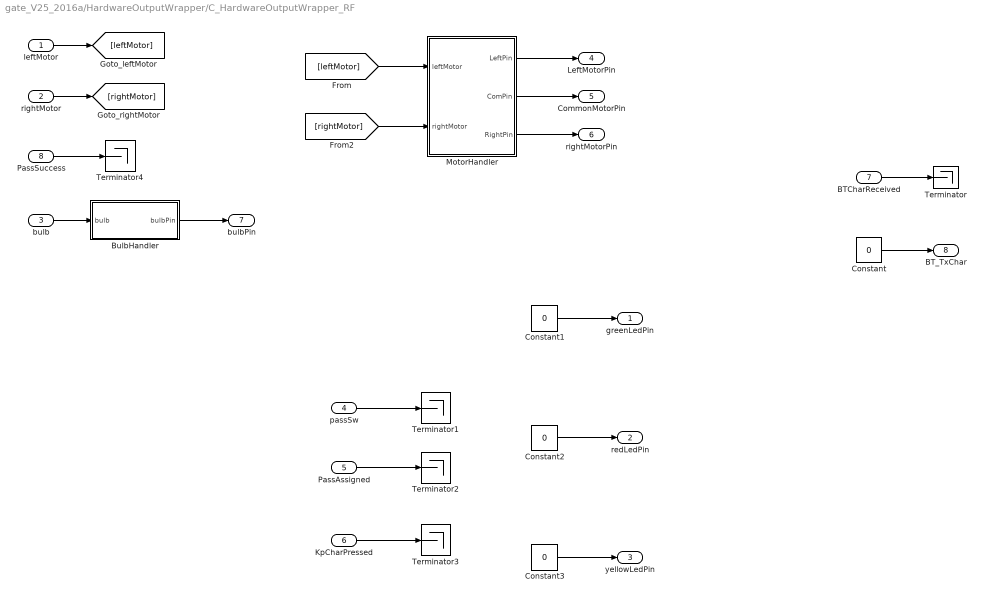
== system gate_V25_2016a/HardwareOutputWrapper/C_HardwareOutputWrapper_RF ==
  leftMotor : Inport
  rightMotor : Inport  Port=2
  bulb : Inport  Port=3
  passSw : Inport  Port=4
  PassAssigned : Inport  Port=5
  KpCharPressed : Inport  Port=6
  BTCharReceived : Inport  Port=7
  PassSuccess : Inport  Port=8
  BulbHandler : Subsystem
  Constant{,1..3} (4 alike) : Constant  Value=0  SampleTime=-1
  MotorHandler : Subsystem
  Terminator{,1..4} (5 alike) : Terminator
  greenLedPin : Outport
  redLedPin : Outport  Port=2
  yellowLedPin : Outport  Port=3
  LeftMotorPin : Outport  Port=4
  CommonMotorPin : Outport  Port=5
  rightMotorPin : Outport  Port=6
  bulbPin : Outport  Port=7
  BT_TxChar : Outport  Port=8
  wires:
  [leftMotor] -> MotorHandler/1(leftMotor)
  [rightMotor] -> MotorHandler/2(rightMotor)
  bulb/1 -> BulbHandler/1(bulb)
  MotorHandler/1(LeftPin) -> LeftMotorPin/1
  MotorHandler/2(ComPin) -> CommonMotorPin/1
  MotorHandler/3(RightPin) -> rightMotorPin/1
  BulbHandler/1(bulbPin) -> bulbPin/1
  leftMotor/1 -> [leftMotor]
  rightMotor/1 -> [rightMotor]
  PassSuccess/1 -> Terminator4/1
  BTCharReceived/1 -> Terminator/1
  Constant/1 -> BT_TxChar/1
  Constant3/1 -> yellowLedPin/1
  Constant2/1 -> redLedPin/1
  Constant1/1 -> greenLedPin/1
  passSw/1 -> Terminator1/1
  PassAssigned/1 -> Terminator2/1
  KpCharPressed/1 -> Terminator3/1

== system gate_V25_2016a/outputPinsBlock/HIL ==
  greenLedPin : Inport
  redLedPin : Inport  Port=2
  yellowLed : Inport  Port=3
  leftMotorPin : Inport  Port=4
  commonMotorPin : Inport  Port=5
  rightMotorPin : Inport  Port=6
  bulbPin : Inport  Port=7
  Digital Output : arduinolib/Digital Output  pinNumber=11  blockPlatform=arduino
  Digital Output1 : arduinolib/Digital Output  pinNumber=12  blockPlatform=arduino
  Digital Output2 : arduinolib/Digital Output  pinNumber=13  blockPlatform=arduino
  S-Function Builder1 : S-Function  InitFcn=try, set_param(gcb,'FunctionName','A2PIN_Lib'), end  FunctionName=A2PIN_Lib  SFunctionModules=A2PIN_Lib_wrapper  SFunctionDeploymentMode=off  EnableBusSupport=off  mask(S-Function Builder){}
      mask help: Simulink:masks:SFunctionBuilder_MD
      mask init: same as gate_V25_2016a/Subsystem/S-Function Builder1
      settings: CopyFcn=set_param(gcbh,'LinkStatus','none')  PreSaveFcn=try, set_param(gcb,'FunctionName','A2PIN_Lib'), end  OpenFcn=sfunctionwizard(gcbh)
      mask Display: plot(val(:,1),val(:,2)),disp(sys), port_label('input',1,'input')
  S-Function Builder2 : S-Function  InitFcn=try, set_param(gcb,'FunctionName','A3PIN_Lib'), end  FunctionName=A3PIN_Lib  SFunctionModules=A3PIN_Lib_wrapper  SFunctionDeploymentMode=off  EnableBusSupport=off  mask(S-Function Builder){}
      mask help: Simulink:masks:SFunctionBuilder_MD
      mask init: same as gate_V25_2016a/Subsystem/S-Function Builder1
      settings: CopyFcn=set_param(gcbh,'LinkStatus','none')  PreSaveFcn=try, set_param(gcb,'FunctionName','A3PIN_Lib'), end  OpenFcn=sfunctionwizard(gcbh)
      mask Display: plot(val(:,1),val(:,2)),disp(sys), port_label('input',1,'input')
  S-Function Builder3 : S-Function  InitFcn=try, set_param(gcb,'FunctionName','A4PIN_Lib'), end  FunctionName=A4PIN_Lib  SFunctionModules=A4PIN_Lib_wrapper  SFunctionDeploymentMode=off  EnableBusSupport=off  mask(S-Function Builder){}
      mask help: Simulink:masks:SFunctionBuilder_MD
      mask init: same as gate_V25_2016a/Subsystem/S-Function Builder1
      settings: CopyFcn=set_param(gcbh,'LinkStatus','none')  PreSaveFcn=try, set_param(gcb,'FunctionName','A4PIN_Lib'), end  OpenFcn=sfunctionwizard(gcbh)
      mask Display: plot(val(:,1),val(:,2)),disp(sys), port_label('input',1,'input')
  S-Function Builder4 : S-Function  InitFcn=try, set_param(gcb,'FunctionName','A5PIN_Lib'), end  FunctionName=A5PIN_Lib  SFunctionModules=A5PIN_Lib_wrapper  SFunctionDeploymentMode=off  EnableBusSupport=off  mask(S-Function Builder){}
      mask help: Simulink:masks:SFunctionBuilder_MD
      mask init: same as gate_V25_2016a/Subsystem/S-Function Builder1
      settings: CopyFcn=set_param(gcbh,'LinkStatus','none')  PreSaveFcn=try, set_param(gcb,'FunctionName','A5PIN_Lib'), end  OpenFcn=sfunctionwizard(gcbh)
      mask Display: plot(val(:,1),val(:,2)),disp(sys), port_label('input',1,'input')
  wires:
  yellowLed/1 -> Digital Output2/1
  leftMotorPin/1 -> S-Function Builder1/1
  commonMotorPin/1 -> S-Function Builder2/1
  rightMotorPin/1 -> S-Function Builder3/1
  bulbPin/1 -> S-Function Builder4/1
  redLedPin/1 -> Digital Output/1
  greenLedPin/1 -> Digital Output1/1

== system gate_V25_2016a/outputPinsBlock/MIL ==
  "leftMotorPin " : Inport
  "commonMotorPin " : Inport  Port=2
  "rightMotorPin " : Inport  Port=3
  greenLedPin : Inport  Port=4
  redLedPin : Inport  Port=5
  yellowLed : Inport  Port=6
  bulbPin : Inport  Port=7
  BT_TxChar : Inport  Port=8
  SimuOutputLimits : Inport  Port=9
  ScopeBlocks : Subsystem  VariantControl=Variant1
  "VerificationBlocks " : Subsystem  VariantControl=Variant2

== system gate_V25_2016a/HardwareInputWrapper/HIL/BluetoothWrapper ==
  S-Function Builder : S-Function  InitFcn=try, set_param(gcb,'FunctionName','BluetoothLib'), end  FunctionName=BluetoothLib  SFunctionModules=BluetoothLib_wrapper  SFunctionDeploymentMode=off  EnableBusSupport=off  mask(S-Function Builder){}
      mask help: Simulink:masks:SFunctionBuilder_MD
      mask init: same as gate_V25_2016a/Subsystem/S-Function Builder1
      settings: CopyFcn=set_param(gcbh,'LinkStatus','none')  PreSaveFcn=try, set_param(gcb,'FunctionName','BluetoothLib'), end  OpenFcn=sfunctionwizard(gcbh)
      mask Display: plot(val(:,1),val(:,2)),disp(sys), port_label('output',1,'BtCharRecieved')
  S-Function Builder1 : S-Function  Commented=on  InitFcn=try, set_param(gcb,'FunctionName','printingBlock'), end  FunctionName=printingBlock  SFunctionModules=printingBlock_wrapper  SFunctionDeploymentMode=off  EnableBusSupport=off  mask(S-Function Builder){}
      mask help: Simulink:masks:SFunctionBuilder_MD
      mask init: same as gate_V25_2016a/Subsystem/S-Function Builder1
      settings: CopyFcn=set_param(gcbh,'LinkStatus','none')  PreSaveFcn=try, set_param(gcb,'FunctionName','printingBlock'), end  OpenFcn=sfunctionwizard(gcbh)
      mask Display: plot(val(:,1),val(:,2)),disp(sys), port_label('input',1,'input'), port_label('input',2,'oldInput')
  Unit Delay : UnitDelay  Commented=on  SampleTime=-1
  bluetoothCharPressed : Outport
  wires:
  S-Function Builder/1 -> S-Function Builder1/1, Unit Delay/1, bluetoothCharPressed/1
  Unit Delay/1 -> S-Function Builder1/2

== system gate_V25_2016a/HardwareInputWrapper/HIL/ButtonsPressed ==
  S-Function Builder1 : S-Function  InitFcn=try, set_param(gcb,'FunctionName','Button_Lib'), end  FunctionName=Button_Lib  SFunctionModules=Button_Lib_wrapper  SFunctionDeploymentMode=off  EnableBusSupport=off  mask(S-Function Builder){}
      mask help: Simulink:masks:SFunctionBuilder_MD
      mask init: same as gate_V25_2016a/Subsystem/S-Function Builder1
      settings: CopyFcn=set_param(gcbh,'LinkStatus','none')  PreSaveFcn=try, set_param(gcb,'FunctionName','Button_Lib'), end  OpenFcn=sfunctionwizard(gcbh)
      mask Display: plot(val(:,1),val(:,2)),disp(sys), port_label('output',1,'RFInput'), port_label('output',2,'passSw')
  RFPressed : Outport
  SWPressed : Outport  Port=2
  wires:
  S-Function Builder1/1 -> RFPressed/1
  S-Function Builder1/2 -> SWPressed/1

== system gate_V25_2016a/HardwareInputWrapper/HIL/KeypadWrapper ==
  KeypadLib : S-Function  InitFcn=try, set_param(gcb,'FunctionName','keypadLib'), end  FunctionName=keypadLib  SFunctionModules=keypadLib_wrapper  SFunctionDeploymentMode=off  EnableBusSupport=off  mask(S-Function Builder){}
      mask help: Simulink:masks:SFunctionBuilder_MD
      mask init: same as gate_V25_2016a/Subsystem/S-Function Builder1
      settings: CopyFcn=set_param(gcbh,'LinkStatus','none')  PreSaveFcn=try, set_param(gcb,'FunctionName','keypadLib'), end  OpenFcn=sfunctionwizard(gcbh)
      mask Display: plot(val(:,1),val(:,2)),disp(sys), port_label('output',1,'charPressed')
  charPressed : Outport
  wires:
  KeypadLib/1 -> charPressed/1

== system gate_V25_2016a/HardwareInputWrapper/HIL/currentSensorWrapperOld ==
  CurrentAnalogIn : Inport
  Add : Sum  Commented=on
  Constant : Constant  Commented=on  Value=0
  Constant1 : Constant  Commented=on
  Divide : Product  Commented=on  Inputs=*/
  Divide1 : Product  Commented=on  Inputs=*/
  MaxAnalog : Constant  Commented=on  Value=65535
  MaxAnalog1 : Constant  Commented=on
  MaxAnalog2 : Constant  Commented=on  Value=600
  MaxVoltage : Constant  Commented=on  Value=5
  Product : Product  Commented=on
  Relational Operator : RelationalOperator  Commented=on  Operator=<=  OutDataTypeStr=boolean
  Slider Gain : simulink/Math Operations/Slider Gain  Commented=on  low=0  gain=1  high=255
  SquareWaveDetector : Stateflow chart  TreatAsAtomicUnit=on
      settings: PermitHierarchicalResolution=ParametersOnly
  Subtract : Sum  Commented=on  Inputs=+-
  Switch : Switch  Commented=on  Criteria=u2 > Threshold
  constantInCurrentEqua : Constant  Commented=on  Value=2.5
  constantInCurrentEqua1 : Constant  Commented=on  Value=0.2
  current : Outport
  wires:
  MaxAnalog/1 -> Divide/2
  Divide/1 -> Product/1
  MaxVoltage/1 -> Product/2
  Product/1 -> Subtract/1
  constantInCurrentEqua/1 -> Subtract/2
  Subtract/1 -> Divide1/1
  constantInCurrentEqua1/1 -> Divide1/2
  Slider Gain/1 -> Divide/1
  Add/1 -> Slider Gain/1
  MaxAnalog1/1 -> Add/1
  MaxAnalog2/1 -> Relational Operator/2
  Relational Operator/1 -> Switch/2
  Constant1/1 -> Switch/3
  Constant/1 -> Switch/1
  CurrentAnalogIn/1 -> SquareWaveDetector/1(CurrentAnalogIn)
  SquareWaveDetector/1(currentValue) -> current/1

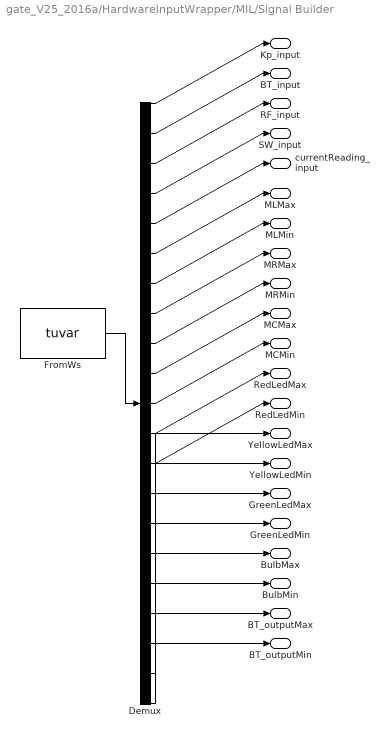
== system gate_V25_2016a/HardwareInputWrapper/MIL/Signal Builder ==
  Demux : Demux  Tag=STV Demux  Outputs=21
  FromWs : FromWorkspace  Tag=STV FromWs  VariableName=tuvar  SampleTime=0
  Kp_input : Outport  Tag=STV Outport
  BT_input : Outport  Tag=STV Outport  Port=2
  RF_input : Outport  Tag=STV Outport  Port=3
  SW_input : Outport  Tag=STV Outport  Port=4
  currentReading_input : Outport  Tag=STV Outport  Port=5
  MLMax : Outport  Tag=STV Outport  Port=6
  MLMin : Outport  Tag=STV Outport  Port=7
  MRMax : Outport  Tag=STV Outport  Port=8
  MRMin : Outport  Tag=STV Outport  Port=9
  MCMax : Outport  Tag=STV Outport  Port=10
  MCMin : Outport  Tag=STV Outport  Port=11
  RedLedMax : Outport  Tag=STV Outport  Port=12
  RedLedMin : Outport  Tag=STV Outport  Port=13
  YellowLedMax : Outport  Tag=STV Outport  Port=14
  YellowLedMin : Outport  Tag=STV Outport  Port=15
  GreenLedMax : Outport  Tag=STV Outport  Port=16
  GreenLedMin : Outport  Tag=STV Outport  Port=17
  BulbMax : Outport  Tag=STV Outport  Port=18
  BulbMin : Outport  Tag=STV Outport  Port=19
  BT_outputMax : Outport  Tag=STV Outport  Port=20
  BT_outputMin : Outport  Tag=STV Outport  Port=21
  wires:
  FromWs/1 -> Demux/1
  Demux/1 -> Kp_input/1
  Demux/2 -> BT_input/1
  Demux/3 -> RF_input/1
  Demux/4 -> SW_input/1
  Demux/5 -> currentReading_input/1
  Demux/6 -> MLMax/1
  Demux/7 -> MLMin/1
  Demux/8 -> MRMax/1
  Demux/9 -> MRMin/1
  Demux/10 -> MCMax/1
  Demux/11 -> MCMin/1
  Demux/12 -> RedLedMax/1
  Demux/13 -> RedLedMin/1
  Demux/14 -> YellowLedMax/1
  Demux/15 -> YellowLedMin/1
  Demux/16 -> GreenLedMax/1
  Demux/17 -> GreenLedMin/1
  Demux/18 -> BulbMax/1
  Demux/19 -> BulbMin/1
  Demux/20 -> BT_outputMax/1
  Demux/21 -> BT_outputMin/1

== system gate_V25_2016a/HardwareOutputWrapper/A_HardwareOutputWrapper_BT_KP_RF/BT_TxHandler ==
  BTCharReceived : Inport
  leftMotor : Inport  Port=2
  rightMotor : Inport  Port=3
  PassSuccess : Inport  Port=4
  BT_TxHandler : Stateflow chart  TreatAsAtomicUnit=on
      settings: PermitHierarchicalResolution=ParametersOnly
  CLOSED : Constant  Value=CLOSED  SampleTime=-1
  CLOSING : Constant  Value=CLOSING  SampleTime=-1
  OPEN : Constant  Value=OPEN  SampleTime=-1
  OPENING : Constant  Value=OPENING  SampleTime=-1
  WRONG_PASSWORD : Constant  Value=WRONG_PASSWORD  SampleTime=-1
  BT_TxChar : Outport
  wires:
  BTCharReceived/1 -> BT_TxHandler/1(BTCharReceived)
  leftMotor/1 -> BT_TxHandler/2(leftMotor)
  rightMotor/1 -> BT_TxHandler/3(rightMotor)
  BT_TxHandler/1(BT_TxChar) -> BT_TxChar/1
  PassSuccess/1 -> BT_TxHandler/4(PassSuccess)
  CLOSED/1 -> BT_TxHandler/5(CLOSED)
  CLOSING/1 -> BT_TxHandler/6(CLOSING)
  OPEN/1 -> BT_TxHandler/7(OPEN)
  OPENING/1 -> BT_TxHandler/8(OPENING)
  WRONG_PASSWORD/1 -> BT_TxHandler/9(WRONG_PASSWORD)

== system gate_V25_2016a/HardwareOutputWrapper/A_HardwareOutputWrapper_BT_KP_RF/BulbHandler ==
  bulb : Inport
  bulbPin : Outport
  wires:
  bulb/1 -> bulbPin/1

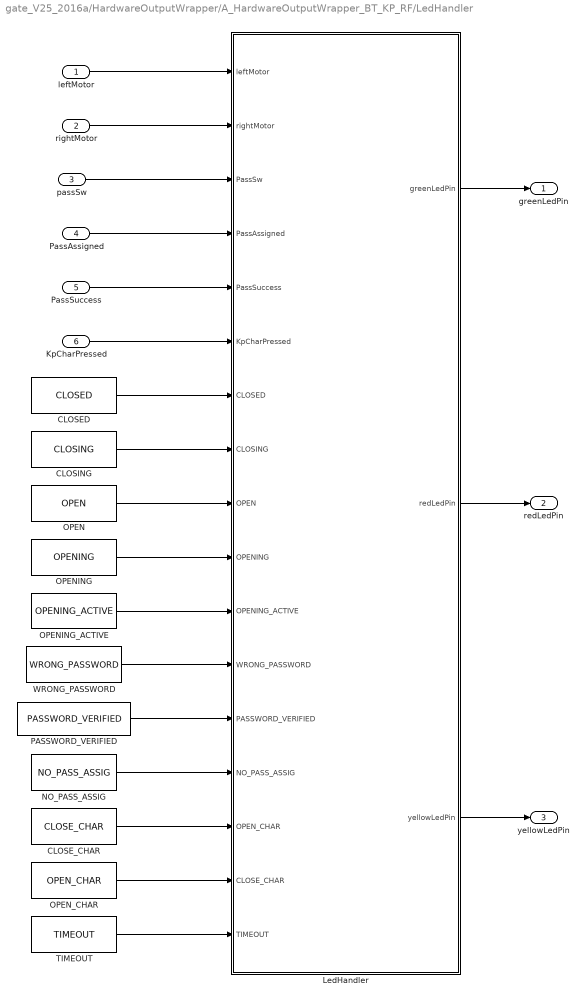
== system gate_V25_2016a/HardwareOutputWrapper/A_HardwareOutputWrapper_BT_KP_RF/LedHandler ==
  leftMotor : Inport
  rightMotor : Inport  Port=2
  passSw : Inport  Port=3
  PassAssigned : Inport  Port=4
  PassSuccess : Inport  Port=5
  KpCharPressed : Inport  Port=6
  CLOSED : Constant  Value=CLOSED  SampleTime=-1
  CLOSE_CHAR : Constant  Value=CLOSE_CHAR  SampleTime=-1
  CLOSING : Constant  Value=CLOSING  SampleTime=-1
  LedHandler : Stateflow chart  TreatAsAtomicUnit=on
      settings: PermitHierarchicalResolution=ParametersOnly
  NO_PASS_ASSIG : Constant  Value=NO_PASS_ASSIG  SampleTime=-1
  OPEN : Constant  Value=OPEN  SampleTime=-1
  OPENING : Constant  Value=OPENING  SampleTime=-1
  OPENING_ACTIVE : Constant  Value=OPENING_ACTIVE  SampleTime=-1
  OPEN_CHAR : Constant  Value=OPEN_CHAR  SampleTime=-1
  PASSWORD_VERIFIED : Constant  Value=PASSWORD_VERIFIED  SampleTime=-1
  TIMEOUT : Constant  Value=TIMEOUT  SampleTime=-1
  WRONG_PASSWORD : Constant  Value=WRONG_PASSWORD  SampleTime=-1
  greenLedPin : Outport
  redLedPin : Outport  Port=2
  yellowLedPin : Outport  Port=3
  wires:
  leftMotor/1 -> LedHandler/1(leftMotor)
  rightMotor/1 -> LedHandler/2(rightMotor)
  LedHandler/1(greenLedPin) -> greenLedPin/1
  LedHandler/2(redLedPin) -> redLedPin/1
  LedHandler/3(yellowLedPin) -> yellowLedPin/1
  passSw/1 -> LedHandler/3(PassSw)
  PassAssigned/1 -> LedHandler/4(PassAssigned)
  PassSuccess/1 -> LedHandler/5(PassSuccess)
  OPENING/1 -> LedHandler/10(OPENING)
  OPEN/1 -> LedHandler/9(OPEN)
  CLOSING/1 -> LedHandler/8(CLOSING)
  CLOSED/1 -> LedHandler/7(CLOSED)
  OPENING_ACTIVE/1 -> LedHandler/11(OPENING_ACTIVE)
  WRONG_PASSWORD/1 -> LedHandler/12(WRONG_PASSWORD)
  PASSWORD_VERIFIED/1 -> LedHandler/13(PASSWORD_VERIFIED)
  NO_PASS_ASSIG/1 -> LedHandler/14(NO_PASS_ASSIG)
  KpCharPressed/1 -> LedHandler/6(KpCharPressed)
  CLOSE_CHAR/1 -> LedHandler/15(OPEN_CHAR)
  OPEN_CHAR/1 -> LedHandler/16(CLOSE_CHAR)
  TIMEOUT/1 -> LedHandler/17(TIMEOUT)

== system gate_V25_2016a/HardwareOutputWrapper/A_HardwareOutputWrapper_BT_KP_RF/MotorHandler ==
  leftMotor : Inport
  rightMotor : Inport  Port=2
  CLOSED : Constant  Value=CLOSED  SampleTime=-1
  CLOSING : Constant  Value=CLOSING  SampleTime=-1
  MotorsHandler : Stateflow chart  TreatAsAtomicUnit=on
      settings: PermitHierarchicalResolution=ParametersOnly
  OPEN : Constant  Value=OPEN  SampleTime=-1
  OPENING : Constant  Value=OPENING  SampleTime=-1
  Unit Delay : UnitDelay  SampleTime=-1
  Unit Delay1 : UnitDelay  SampleTime=-1
  LeftPin : Outport
  ComPin : Outport  Port=2
  RightPin : Outport  Port=3
  wires:
  leftMotor/1 -> Unit Delay/1, MotorsHandler/1(leftMotor)
  Unit Delay/1 -> MotorsHandler/2(oldLeft)
  rightMotor/1 -> Unit Delay1/1, MotorsHandler/3(rightMotor)
  Unit Delay1/1 -> MotorsHandler/4(oldRight)
  CLOSED/1 -> MotorsHandler/5(CLOSED)
  CLOSING/1 -> MotorsHandler/6(CLOSING)
  OPEN/1 -> MotorsHandler/7(OPEN)
  OPENING/1 -> MotorsHandler/8(OPENING)
  MotorsHandler/1(LeftPin) -> LeftPin/1
  MotorsHandler/2(ComPin) -> ComPin/1
  MotorsHandler/3(RightPin) -> RightPin/1

== system gate_V25_2016a/HardwareOutputWrapper/B_HardwareOutputWrapper_KP_RF/BulbHandler ==
  bulb : Inport
  bulbPin : Outport
  wires:
  bulb/1 -> bulbPin/1
